simulink model "Pong"  (Simulink 7.0)
settings: Solver=ode4  StartTime=0.0  StopTime=inf  FixedStep=0.001  RelTol=1e-3
undefined symbols (not defined in the file): HIL, qc_get_step_size
libraries: simulink x6, quarc_library x4, vrlib x1
settings Model: Creator=RSamra  LastModifiedBy=colinlea  SimulationMode=external  ExtModeTrigDuration=10000
settings SolverCC: PositivePriorityOrder=on
settings DebuggingCC: MultiTaskDSMMsg=warning  MultiTaskCondExecSysMsg=none  StrictBusMsg=None
settings HardwareCC: TargetHWDeviceType=32-bit Generic
settings RTWCC: SystemTargetFile=quarc_windows.tlc  TemplateMakefile=quarc_default_tmf  Description=QuaRC Win32 Target  ProcessScript=quarc_windows_make_rtw_hook  IncludeERTFirstTime=on
settings STFCustomTargetCC: TargetFcnLib=ansi_tfl_tmw.mat  TargetPreCompLibLocation=C:\DOCUME~1\ALLUSE~1\APPLIC~1\QuaRC\lib\2007b\windows\release  GenFloatMathFcnCalls=ANSI_C  SystemTargetFile=quarc_windows.tlc
settings GRTTargetCC: TargetFcnLib=ansi_tfl_tmw.mat  TargetPreCompLibLocation=C:\DOCUME~1\ALLUSE~1\APPLIC~1\QuaRC\lib\2007b\windows\release  CompOptLevelCompliant=off  MatFileLogging=off  ExtMode=on  ExtModeMexFile=quarc_comm

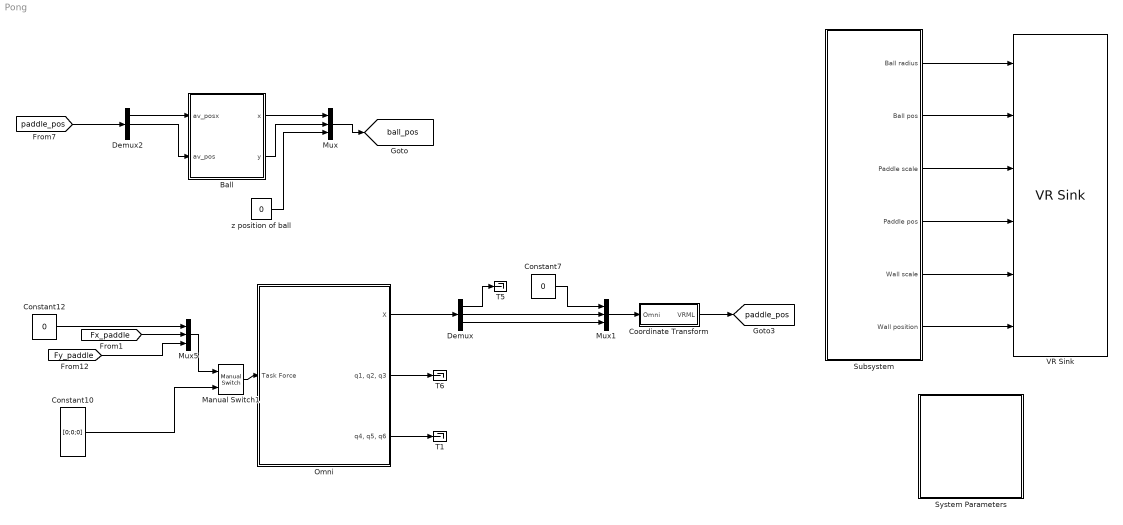
== system Pong ==
  Ball : Subsystem
  Constant10 : Constant  Value=[0;0;0]  VectorParams1D=off  OutDataType=sfix(16)  OutScaling=2^0  SampleTime=0
  Constant12 : Constant  Value=0  VectorParams1D=off  OutDataType=sfix(16)  OutScaling=2^0  SampleTime=0
  Constant7 : Constant  Value=0  VectorParams1D=off  OutDataType=sfix(16)  OutScaling=2^0  SampleTime=0
  Coordinate Transform : Subsystem
  Demux : Demux  Outputs=3
  Demux2 : Demux  Outputs=3
  Manual Switch1 : simulink/Signal Routing/Manual Switch  SystemSampleTime=-1  sw=1  action=0  varsize=off
  Mux : Mux  Inputs=3
  Mux1 : Mux  Inputs=3
  Mux5 : Mux  Inputs=3
  Omni : Subsystem
  Subsystem : Subsystem
  System Parameters : Subsystem
  T1 : Terminator
  T5 : Terminator
  T6 : Terminator
  VR Sink : vrlib/VR Sink  SampleTime=.1  ViewEnable=on  RemoteChange=off  RemoteView=on  FieldsWritten=Ball.scale.3.1.double#Ball.translation.3.1.double#Paddle.scale.3.1.double#Paddle.translation.3.1.double#Walls.scale.3.1.double#Walls.translation.3.1.double  WorldFileName=Pong.WRL  AutoView=on  VideoDimensions=[]  FigureProperties="{'Position', 'Name', 'Viewpoint', 'CameraBound', 'CameraDirection', 'CameraPosition', 'CameraUpVector', 'ZoomFactor', 'Antialiasing', 'Headlight', 'Lighting', 'NavPanel', 'StatusBar', 'ToolBar', 'Textures', 'Transparency', 'Wireframe', 'NavZones', 'NavMode', 'NavSpeed', 'Record2DCompressMethod', 'Record2DCompressQuality', 'Record2D', 'Record2DFileName', 'Record2DFPS'; [-3.0000000000000000e+000  1.1900000000000000e+002  5.7600000000000000e+002  3.8000000000000000e+002], '', '_untitled_1', 'on', [0.0000000000000000e+000  0.0000000000000000e+000 -1.0000000000000000e+000], [0.0000000000000000e+000  0.0000000000000000e+000  0.0000000000000000e+000], [0.0000000000000000e+000  1.0000000000000000e+000  0.0000000000000000e+000], [1.0000000000000000e+000], 'off', 'on', 'on', 'halfbar', 'off', 'on', 'on', 'on', 'off', 'off', 'fly', 'normal', 'auto', [7.5000000000000000e+001], 'off', '%f_anim_%n.avi', [1.5000000000000000e+001]}"
  z position of ball : Constant  Value=0  VectorParams1D=off  OutDataType=sfix(16)  OutScaling=2^0  SampleTime=0
  tag scope: ball_pos=global, paddle_pos=global
  wires:
  Mux/1 -> [ball_pos]
  z position of ball/1 -> Mux/3
  Ball/1(x) -> Mux/1
  Ball/2(y) -> Mux/2
  Constant7/1 -> Mux1/1
  Mux1/1 -> Coordinate Transform/1(Omni)
  Coordinate Transform/1("VRML ") -> [paddle_pos]
  Demux/1 -> T5/1
  Subsystem/1(Ball radius) -> VR Sink/1
  Subsystem/3(Paddle scale) -> VR Sink/3
  Subsystem/5(Wall scale) -> VR Sink/5
  Subsystem/6(Wall position) -> VR Sink/6
  [paddle_pos] -> Demux2/1
  Subsystem/4(Paddle pos) -> VR Sink/4
  Subsystem/2(Ball pos) -> VR Sink/2
  Constant10/1 -> Manual Switch1/2
  Constant12/1 -> Mux5/1
  Mux5/1 -> Manual Switch1/1
  [Fx_paddle] -> Mux5/2
  [Fy_paddle] -> Mux5/3
  Demux2/2 -> Ball/2(av_pos)
  Demux/2 -> Mux1/2
  Demux/3 -> Mux1/3
  Demux2/1 -> Ball/1(av_posx)
  Omni/1(X) -> Demux/1
  Omni/2("q1, q2, q3") -> T6/1
  Omni/3("q4, q5, q6") -> T1/1
  Manual Switch1/1 -> Omni/1(Task Force)

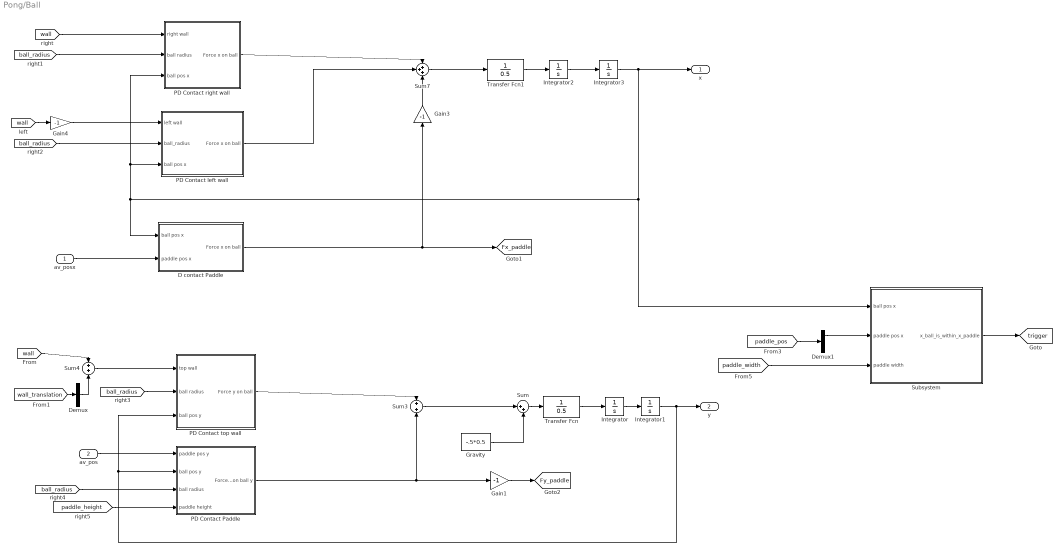
== system Pong/Ball ==
  av_posx : Inport  OutDataType=sfix(16)  OutScaling=2^0
  av_pos : Inport  Port=2  OutDataType=sfix(16)  OutScaling=2^0
  D contact Paddle : Subsystem
  Demux : Demux  Outputs=3
  Demux1 : Demux  Outputs=3
  Gain1 : Gain  Gain=-1  ParameterDataType=sfix(16)  ParameterScaling=2^0  OutDataType=sfix(16)  OutScaling=2^0
  Gain3 : Gain  Orientation=up  Gain=-1  ParameterDataType=sfix(16)  ParameterScaling=2^0  OutDataType=sfix(16)  OutScaling=2^0
  Gain4 : Gain  Gain=-1  ParameterDataType=sfix(16)  ParameterScaling=2^0  OutDataType=sfix(16)  OutScaling=2^0
  Gravity : Constant  Value=-.5*0.5  OutDataType=sfix(16)  OutScaling=2^0  SampleTime=0
  Integrator{,1..3} (4 alike) : Integrator
  PD Contact Paddle : Subsystem
  PD Contact left wall : Subsystem
  PD Contact right wall : Subsystem
  PD Contact top wall : Subsystem
  Subsystem : Subsystem
  Sum : Sum  Inputs=|++  OutDataType=sfix(16)  OutScaling=2^0
  Sum3 : Sum  OutDataType=sfix(16)  OutScaling=2^0
  Sum4 : Sum  OutDataType=sfix(16)  OutScaling=2^0
  Sum7 : Sum  Inputs=+++  OutDataType=sfix(16)  OutScaling=2^0
  Transfer Fcn : TransferFcn  Denominator=[0.5]
  Transfer Fcn1 : TransferFcn  Denominator=[0.5]
  x : Outport
  y : Outport  Port=2
  tag scope: Fx_paddle=global, Fy_paddle=global, trigger=global
  wires:
  Transfer Fcn/1 -> Integrator/1
  Integrator/1 -> Integrator1/1
  Sum/1 -> Transfer Fcn/1
  Gravity/1 -> Sum/2
  Integrator1/1 -> y/1, PD Contact top wall/3(ball pos y), PD Contact Paddle/2(ball pos y)
  PD Contact top wall/1("Force y on ball ") -> Sum3/1
  PD Contact Paddle/1(Force on ball y) -> Sum3/2, Gain1/1
  Sum3/1 -> Sum/1
  Transfer Fcn1/1 -> Integrator2/1
  Integrator2/1 -> Integrator3/1
  Integrator3/1 -> x/1, PD Contact left wall/3(ball pos x), PD Contact right wall/3(ball pos x), D contact Paddle/1(ball pos x), Subsystem/1(ball pos x)
  PD Contact right wall/1(Force x on ball) -> Sum7/1
  PD Contact left wall/1(Force x on ball) -> Sum7/2
  Sum7/1 -> Transfer Fcn1/1
  [wall] -> Sum4/1
  [wall] -> Gain4/1
  [wall] -> PD Contact right wall/1(right wall)
  Gain4/1 -> PD Contact left wall/1(left wall)
  [wall_translation] -> Demux/1
  [paddle_width] -> Subsystem/3(paddle width)
  Subsystem/1(x_ball_is_within_x_paddle) -> [trigger]
  [ball_radius] -> PD Contact left wall/2(ball_radius)
  Gain1/1 -> [Fy_paddle]
  Demux/2 -> Sum4/2
  [ball_radius] -> PD Contact top wall/2(ball radius)
  Sum4/1 -> PD Contact top wall/1(top wall)
  av_pos/1 -> PD Contact Paddle/1(paddle pos y)
  [ball_radius] -> PD Contact Paddle/3(ball radius)
  [paddle_height] -> PD Contact Paddle/4(paddle height)
  [ball_radius] -> PD Contact right wall/2(ball radius)
  Gain3/1 -> Sum7/3
  av_posx/1 -> D contact Paddle/2(paddle pos x)
  D contact Paddle/1("Force x on ball ") -> Gain3/1, [Fx_paddle]
  [paddle_pos] -> Demux1/1
  Demux1/1 -> Subsystem/2(paddle pos x)

== system Pong/Coordinate Transform ==
  Omni : Inport  Orientation=down
  Demux1 : Demux  Outputs=3
  Mux : Mux  Inputs=3
  "VRML " : Outport
  wires:
  Omni/1 -> Demux1/1
  Mux/1 -> "VRML "/1
  Demux1/1 -> Mux/3
  Demux1/3 -> Mux/2
  Demux1/2 -> Mux/1

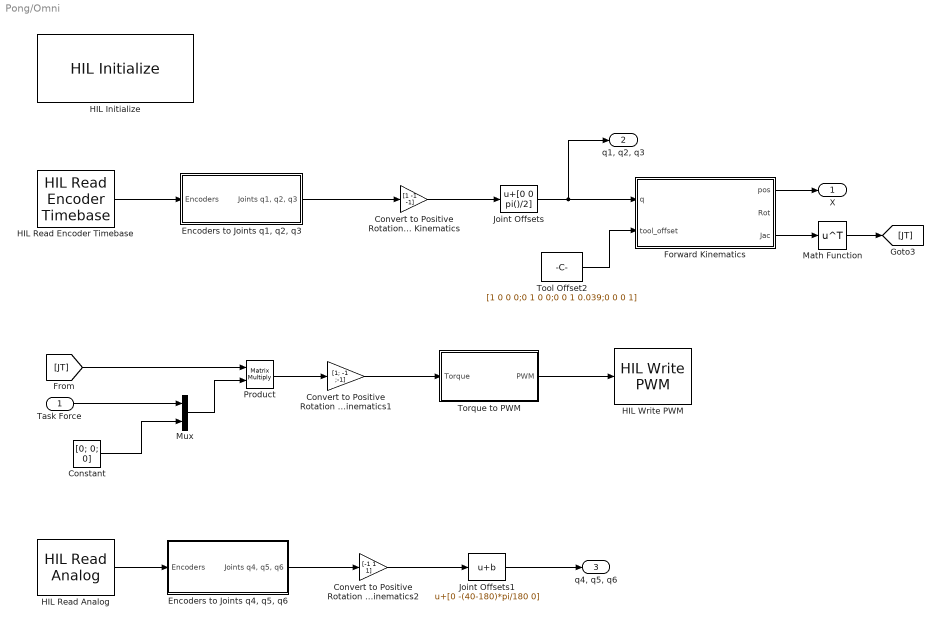
== system Pong/Omni ==
  Task Force : Inport
  Constant : Constant  Value=[0; 0; 0]  VectorParams1D=off  OutDataType=sfix(16)  OutScaling=2^0
  Convert to Positive Rotation Convension Used in Kinematics : Gain  Gain=[1 -1 -1]  ParameterDataType=sfix(16)  ParameterScaling=2^0  OutDataType=sfix(16)  OutScaling=2^0
  Convert to Positive Rotation Convension Used in Kinematics1 : Gain  Gain=[1; -1 ;-1]  ParameterDataType=sfix(16)  ParameterScaling=2^0  OutDataType=sfix(16)  OutScaling=2^0
  Convert to Positive Rotation Convension Used in Kinematics2 : Gain  Gain=[-1 1 1]  ParameterDataType=sfix(16)  ParameterScaling=2^0  OutDataType=sfix(16)  OutScaling=2^0
  "Encoders to Joints q1, q2, q3" : Subsystem
  "Encoders to Joints q4, q5, q6" : Subsystem
  "Forward Kinematics " : Stateflow chart
  HIL Initialize : quarc_library/Data Acquisition/Generic/Configuration/HIL Initialize  object_name=HIL-1  board_type=phantom_omni  board_number=0  active=on  hardware_clocks=[]  clock_modes=[]  set_clock_params_at_start=off  set_clock_params_at_switch_in=off  analog_input_channels=0:1  analog_input_maximums=10  analog_input_minimums=-10  set_analog_input_params_at_start=off  set_analog_input_params_at_switch_in=off  analog_output_channels=[]  analog_output_maximums=[]  analog_output_minimums=[]  initial_analog_outputs=[]  final_analog_outputs=[]  watchdog_analog_outputs=0  set_analog_output_params_at_start=off  set_analog_output_params_at_switch_in=off  set_analog_outputs_at_start=off  set_analog_outputs_at_switch_in=off  set_analog_outputs_at_terminate=off  set_analog_outputs_at_switch_out=off  set_analog_outputs_on_watchdog=off  digital_input_channels=[]  digital_output_channels=[]  initial_digital_outputs=[]  final_digital_outputs=[]  watchdog_digital_outputs=0  set_digital_outputs_at_start=off  set_digital_outputs_at_switch_in=off  set_digital_outputs_at_terminate=off  set_digital_outputs_at_switch_out=off  set_digital_outputs_on_watchdog=off  encoder_channels=0:2  quadrature=[]  encoder_filter_frequency=[]  initial_encoder_counts=0  set_encoder_params_at_start=off  set_encoder_params_at_switch_in=off  set_encoder_counts_at_start=off  set_encoder_counts_at_switch_in=off  pwm_channels=0:2  pwm_modes=[]  pwm_frequency=[]  initial_pwm_outputs=0  final_pwm_outputs=0  watchdog_pwm_outputs=0  set_pwm_params_at_start=off  set_pwm_params_at_switch_in=off  set_pwm_outputs_at_start=on  set_pwm_outputs_at_switch_in=off  set_pwm_outputs_at_terminate=on  set_pwm_outputs_at_switch_out=off  set_pwm_outputs_on_watchdog=off  other_output_channels=[]  initial_other_outputs=[]  final_other_outputs=[]  watchdog_other_outputs=0  set_other_outputs_at_start=off  set_other_outputs_at_switch_in=off  set_other_outputs_at_terminate=off  set_other_outputs_at_switch_out=off  set_other_outputs_on_watchdog=off
  HIL Read Analog : quarc_library/Data Acquisition/Generic/Immediate I//O/HIL Read Analog  object_name=HIL-1  channels=[0:2]  sample_time=qc_get_step_size  active=on  vector_output=on
  HIL Read Encoder Timebase : quarc_library/Data Acquisition/Generic/Timebases/HIL Read Encoder Timebase  object_name=HIL-1  clock=0  channels=0:2  samples_in_buffer=max(ceil(1/qc_get_step_size), 1)  active=on  vector_output=on  data_type_mode=Inherit via back propagation  data_type=double
  HIL Write PWM : quarc_library/Data Acquisition/Generic/Immediate I//O/HIL Write PWM  object_name=HIL-1  channels=0:2  sample_time=-1  active=off  vector_input=on
      settings: AttributesFormatString=(%<object_name>)
  Joint Offsets : Bias  Bias=[0 0 pi()/2]
  Joint Offsets1 : Bias  Bias=[0 -(40-180)*pi/180 0]  SaturateOnIntegerOverflow=on
  Math Function : Math  Operator=transpose  OutDataType=sfix(16)  OutScaling=2^0  SaturateOnIntegerOverflow=on
  Mux : Mux  Inputs=2
  Product : Product  Multiplication=Matrix(*)  OutDataType=sfix(16)  OutScaling=2^0  RndMeth=Zero
  Tool Offset2 : Constant  Value=[1 0 0 0;0 1 0 0;0 0 1 0.039;0 0 0 1]  VectorParams1D=off  OutDataType=sfix(16)  OutScaling=2^0
  Torque to PWM : Subsystem
  X : Outport
  "q1, q2, q3" : Outport  Port=2
  "q4, q5, q6" : Outport  Port=3
  wires:
  Tool Offset2/1 -> "Forward Kinematics "/2(tool_offset)
  Math Function/1 -> [JT]
  "Forward Kinematics "/3(Jac) -> Math Function/1
  [JT] -> Product/1
  Torque to PWM/1(PWM) -> HIL Write PWM/1
  "Forward Kinematics "/1(pos) -> X/1
  Constant/1 -> Mux/2
  Task Force/1 -> Mux/1
  Mux/1 -> Product/2
  "Encoders to Joints q1, q2, q3"/1("Joints q1, q2, q3") -> Convert to Positive Rotation Convension Used in Kinematics/1
  Convert to Positive Rotation Convension Used in Kinematics/1 -> Joint Offsets/1
  Convert to Positive Rotation Convension Used in Kinematics1/1 -> Torque to PWM/1(Torque)
  Product/1 -> Convert to Positive Rotation Convension Used in Kinematics1/1
  Joint Offsets/1 -> "Forward Kinematics "/1(q), "q1, q2, q3"/1
  HIL Read Encoder Timebase/1 -> "Encoders to Joints q1, q2, q3"/1(Encoders)
  HIL Read Analog/1 -> "Encoders to Joints q4, q5, q6"/1(Encoders)
  Convert to Positive Rotation Convension Used in Kinematics2/1 -> Joint Offsets1/1
  "Encoders to Joints q4, q5, q6"/1("Joints q4, q5, q6") -> Convert to Positive Rotation Convension Used in Kinematics2/1
  Joint Offsets1/1 -> "q4, q5, q6"/1

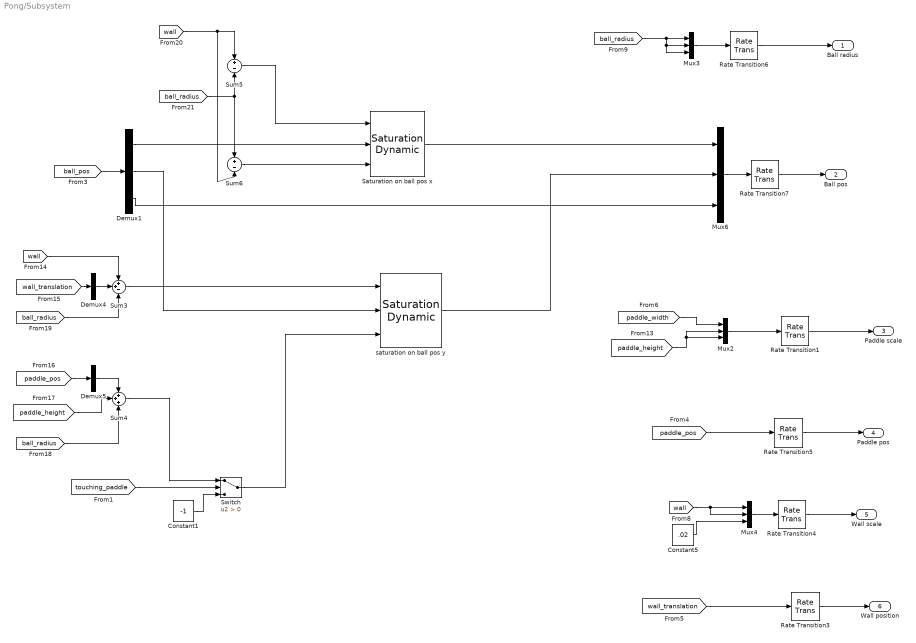
== system Pong/Subsystem ==
  Constant1 : Constant  Value=-1  OutDataType=sfix(16)  OutScaling=2^0
  Constant5 : Constant  Value=.02  VectorParams1D=off  OutDataType=sfix(16)  OutScaling=2^0  SampleTime=0
  Demux1 : Demux  Outputs=3
  Demux4 : Demux  Outputs=3
  Demux5 : Demux  Outputs=3
  Mux{2..4,6} (4 alike) : Mux  Inputs=3
  Rate Transition{1,3..7} (6 alike) : RateTransition
  Saturation on ball pos x : simulink/Discontinuities/Saturation Dynamic  SystemSampleTime=-1  OutMin=[]  OutMax=[]  OutDataTypeStr=Inherit: Same as second input  OutDataType=sfix(16)  OutScaling=2^-10  DoSatur=off
  Sum3 : Sum  Inputs=++-  OutDataType=sfix(16)  OutScaling=2^0
  Sum4 : Sum  Inputs=+++  OutDataType=sfix(16)  OutScaling=2^0
  Sum5 : Sum  Inputs=+-  OutDataType=sfix(16)  OutScaling=2^0
  Sum6 : Sum  Inputs=+-  OutDataType=sfix(16)  OutScaling=2^0
  Switch : Switch  Criteria=u2 > Threshold
  saturation on ball pos y : simulink/Discontinuities/Saturation Dynamic  SystemSampleTime=-1  OutMin=[]  OutMax=[]  OutDataTypeStr=Inherit: Same as second input  OutDataType=sfix(16)  OutScaling=2^-10  DoSatur=off
  Ball radius : Outport
  Ball pos : Outport  Port=2
  Paddle scale : Outport  Port=3
  Paddle pos : Outport  Port=4
  Wall scale : Outport  Port=5
  Wall position : Outport  Port=6
  wires:
  [paddle_width] -> Mux2/1
  [paddle_height] -> Mux2/2, Mux2/3
  [ball_radius] -> Mux3/1, Mux3/2, Mux3/3
  Mux4/1 -> Rate Transition4/1
  Mux2/1 -> Rate Transition1/1
  Mux3/1 -> Rate Transition6/1
  [wall] -> Mux4/1, Mux4/2
  Constant5/1 -> Mux4/3
  [paddle_pos] -> Rate Transition5/1
  [wall_translation] -> Rate Transition3/1
  [ball_pos] -> Demux1/1
  Mux6/1 -> Rate Transition7/1
  Demux1/3 -> Mux6/3
  Demux1/2 -> saturation on ball pos y/2
  saturation on ball pos y/1 -> Mux6/2
  [wall_translation] -> Demux4/1
  [wall] -> Sum3/1
  Demux4/2 -> Sum3/2
  Sum3/1 -> saturation on ball pos y/1
  [paddle_pos] -> Demux5/1
  Demux5/2 -> Sum4/1
  [paddle_height] -> Sum4/2
  [ball_radius] -> Sum4/3
  [ball_radius] -> Sum3/3
  Demux1/1 -> Saturation on ball pos x/2
  Saturation on ball pos x/1 -> Mux6/1
  [wall] -> Sum5/1, Sum6/2
  [ball_radius] -> Sum5/2, Sum6/1
  Sum5/1 -> Saturation on ball pos x/1
  Rate Transition6/1 -> Ball radius/1
  Rate Transition7/1 -> Ball pos/1
  Rate Transition1/1 -> Paddle scale/1
  Rate Transition5/1 -> Paddle pos/1
  Rate Transition4/1 -> Wall scale/1
  Rate Transition3/1 -> Wall position/1
  Sum6/1 -> Saturation on ball pos x/3
  Switch/1 -> saturation on ball pos y/3
  [touching_paddle] -> Switch/2
  Sum4/1 -> Switch/1
  Constant1/1 -> Switch/3

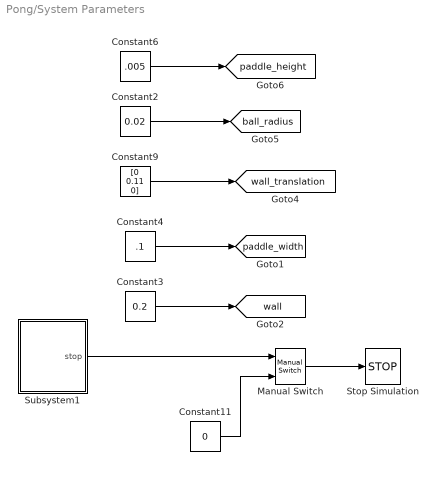
== system Pong/System Parameters ==
  Constant11 : Constant  Value=0  OutDataType=sfix(16)  OutScaling=2^0  SampleTime=0
  Constant2 : Constant  Value=0.02  VectorParams1D=off  OutDataType=sfix(16)  OutScaling=2^0
  Constant3 : Constant  Value=0.2  OutDataType=sfix(16)  OutScaling=2^0  SampleTime=0
  Constant4 : Constant  Value=.1  VectorParams1D=off  OutDataType=sfix(16)  OutScaling=2^0  SampleTime=0
  Constant6 : Constant  Value=.005  VectorParams1D=off  OutDataType=sfix(16)  OutScaling=2^0  SampleTime=0
  Constant9 : Constant  Value=[0 0.11 0]  VectorParams1D=off  OutDataType=sfix(16)  OutScaling=2^0  SampleTime=0
  Manual Switch : simulink/Signal Routing/Manual Switch  SystemSampleTime=-1  sw=1  action=0  varsize=off
  Stop Simulation : Stop
  Subsystem1 : Subsystem
  tag scope: ball_radius=global, paddle_height=global, paddle_width=global, wall=global, wall_translation=global
  wires:
  Constant4/1 -> [paddle_width]
  Constant3/1 -> [wall]
  Constant9/1 -> [wall_translation]
  Manual Switch/1 -> Stop Simulation/1
  Subsystem1/1(stop) -> Manual Switch/1
  Constant11/1 -> Manual Switch/2
  Constant2/1 -> [ball_radius]
  Constant6/1 -> [paddle_height]

== system Pong/Ball/D contact Paddle ==
  ball pos x : Inport
  paddle pos x : Inport  Port=2
  Compare To Constant1 : simulink/Logic and Bit Operations/Compare To Constant  SystemSampleTime=-1  relop=~=  const=0  LogicOutDataTypeMode=uint8  ZeroCross=off
  Logical Operator2 : Logic  AllPortsSameDT=off  OutDataTypeMode=boolean
  Subsystem5 : Subsystem
  Sum10 : Sum  Inputs=-+  OutDataType=sfix(16)  OutScaling=2^0
  Switch4 : Switch  Criteria=u2 > Threshold
  non contact Force4 : Constant  Value=0  VectorParams1D=off  OutDataType=sfix(16)  OutScaling=2^0  SampleTime=0
  "Force x on ball " : Outport
  wires:
  Sum10/1 -> Compare To Constant1/1, Subsystem5/1(In1)
  Compare To Constant1/1 -> Logical Operator2/1
  Logical Operator2/1 -> Switch4/2
  non contact Force4/1 -> Switch4/3
  Subsystem5/1(Fball) -> Switch4/1
  ball pos x/1 -> Sum10/1
  Switch4/1 -> "Force x on ball "/1
  paddle pos x/1 -> Sum10/2
  [touching_paddle] -> Logical Operator2/2

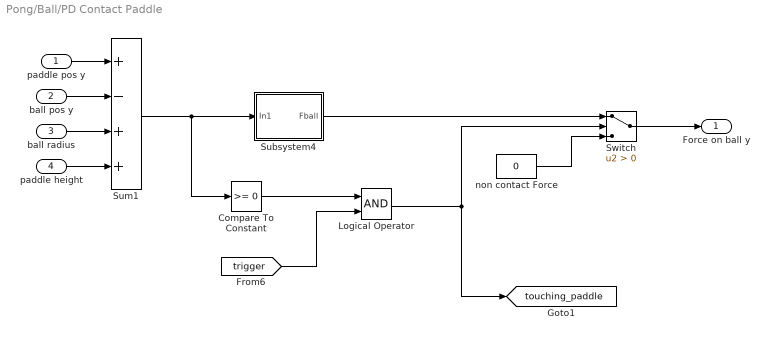
== system Pong/Ball/PD Contact Paddle ==
  paddle pos y : Inport
  ball pos y : Inport  Port=2
  ball radius : Inport  Port=3
  paddle height : Inport  Port=4
  Compare To Constant : simulink/Logic and Bit Operations/Compare To Constant  SystemSampleTime=-1  relop=>=  const=0  LogicOutDataTypeMode=uint8  ZeroCross=off
  Logical Operator : Logic  AllPortsSameDT=off  OutDataTypeMode=boolean
  Subsystem4 : Subsystem
  Sum1 : Sum  Inputs=+-++  OutDataType=sfix(16)  OutScaling=2^0
  Switch : Switch  Criteria=u2 > Threshold
  non contact Force : Constant  Value=0  VectorParams1D=off  OutDataType=sfix(16)  OutScaling=2^0  SampleTime=0
  Force on ball y : Outport
  tag scope: touching_paddle=global
  wires:
  Sum1/1 -> Subsystem4/1(In1), Compare To Constant/1
  Compare To Constant/1 -> Logical Operator/1
  [trigger] -> Logical Operator/2
  Logical Operator/1 -> Switch/2, [touching_paddle]
  Subsystem4/1(Fball) -> Switch/1
  non contact Force/1 -> Switch/3
  ball pos y/1 -> Sum1/2
  paddle pos y/1 -> Sum1/1
  Switch/1 -> Force on ball y/1
  ball radius/1 -> Sum1/3
  paddle height/1 -> Sum1/4

== system Pong/Ball/PD Contact left wall ==
  left wall : Inport
  ball_radius : Inport  Port=2
  ball pos x : Inport  Port=3
  Subsystem1 : Subsystem
  Sum5 : Sum  Inputs=++-  OutDataType=sfix(16)  OutScaling=2^0
  Switch2 : Switch
  non contact Force2 : Constant  Value=0  VectorParams1D=off  OutDataType=sfix(16)  OutScaling=2^0  SampleTime=0
  Force x on ball : Outport
  wires:
  non contact Force2/1 -> Switch2/3
  Subsystem1/1(Fball) -> Switch2/1
  Sum5/1 -> Subsystem1/1(In1), Switch2/2
  ball_radius/1 -> Sum5/2
  left wall/1 -> Sum5/1
  Switch2/1 -> Force x on ball/1
  ball pos x/1 -> Sum5/3

== system Pong/Ball/PD Contact right wall ==
  right wall : Inport
  ball radius : Inport  Port=2
  ball pos x : Inport  Port=3
  Subsystem2 : Subsystem
  Sum6 : Sum  Inputs=+--  OutDataType=sfix(16)  OutScaling=2^0
  Switch3 : Switch
  non contact Force3 : Constant  Value=0  VectorParams1D=off  OutDataType=sfix(16)  OutScaling=2^0  SampleTime=0
  Force x on ball : Outport
  wires:
  non contact Force3/1 -> Switch3/1
  Sum6/1 -> Switch3/2, Subsystem2/1(In1)
  Subsystem2/1(Fball) -> Switch3/3
  Switch3/1 -> Force x on ball/1
  right wall/1 -> Sum6/1
  ball radius/1 -> Sum6/2
  ball pos x/1 -> Sum6/3

== system Pong/Ball/PD Contact top wall ==
  top wall : Inport
  ball radius : Inport  Port=2
  ball pos y : Inport  Port=3
  Subsystem3 : Subsystem
  Sum2 : Sum  Inputs=+--  OutDataType=sfix(16)  OutScaling=2^0
  Switch1 : Switch
  non contact Force1 : Constant  Value=0  VectorParams1D=off  OutDataType=sfix(16)  OutScaling=2^0  SampleTime=0
  "Force y on ball " : Outport
  wires:
  Subsystem3/1(Fball) -> Switch1/3
  non contact Force1/1 -> Switch1/1
  ball pos y/1 -> Sum2/3
  Switch1/1 -> "Force y on ball "/1
  top wall/1 -> Sum2/1
  ball radius/1 -> Sum2/2
  Sum2/1 -> Subsystem3/1(In1), Switch1/2

== system Pong/Ball/Subsystem ==
  ball pos x : Inport
  paddle pos x : Inport  Port=2
  paddle width : Inport  Port=3
  Logical Operator1 : Logic  AllPortsSameDT=off  OutDataTypeMode=boolean
  Relational Operator : RelationalOperator  Operator=<=  LogicOutDataTypeMode=boolean
  Relational Operator1 : RelationalOperator  LogicOutDataTypeMode=boolean
  Sum8 : Sum  OutDataType=sfix(16)  OutScaling=2^0
  Sum9 : Sum  Inputs=-+  OutDataType=sfix(16)  OutScaling=2^0
  x_ball_is_within_x_paddle : Outport
  wires:
  Sum8/1 -> Relational Operator/2
  Sum9/1 -> Relational Operator1/2
  Relational Operator/1 -> Logical Operator1/1
  Relational Operator1/1 -> Logical Operator1/2
  ball pos x/1 -> Relational Operator/1, Relational Operator1/1
  paddle pos x/1 -> Sum8/1, Sum9/2
  paddle width/1 -> Sum8/2, Sum9/1
  Logical Operator1/1 -> x_ball_is_within_x_paddle/1

== system Pong/Omni/Encoders to Joints q1, q2, q3 ==
  Encoders : Inport
  Bias1 : Bias  Bias=[0 -659 -910]
  Embedded MATLAB Function : Stateflow chart
  Encoder : Gain  Gain=2*pi/2048  ParameterDataType=sfix(16)  ParameterScaling=2^0  OutDataType=sfix(16)  OutScaling=2^0
  Gear Ratio : Gain  Gain=1./[7.461 -7.519 7.529]  ParameterDataType=sfix(16)  ParameterScaling=2^0  OutDataType=sfix(16)  OutScaling=2^0
  "Joints q1, q2, q3" : Outport
  wires:
  Embedded MATLAB Function/1(q) -> "Joints q1, q2, q3"/1
  Encoders/1 -> Bias1/1
  Encoder/1 -> Gear Ratio/1
  Gear Ratio/1 -> Embedded MATLAB Function/1(m)
  Bias1/1 -> Encoder/1

== system Pong/Omni/Encoders to Joints q4, q5, q6 ==
  Encoders : Inport
  Bias1 : Bias  Bias=[-2048 -2654 -2048]
  Gain2 : Gain  Gain=[2*pi()/4915 2*pi()/4096 2*pi()/4915]  ParameterDataType=sfix(16)  ParameterScaling=2^0  OutDataType=sfix(16)  OutScaling=2^0
  "Joints q4, q5, q6" : Outport
  wires:
  Bias1/1 -> Gain2/1
  Encoders/1 -> Bias1/1
  Gain2/1 -> "Joints q4, q5, q6"/1

== system Pong/Omni/Torque to PWM ==
  Torque : Inport
  Gear Ratio1 : Gain  Gain=1./[7.461 -7.519 7.529]  ParameterDataType=sfix(16)  ParameterScaling=2^0  OutDataType=sfix(16)  OutScaling=2^0
  Joint Torque to Motor Torque : Stateflow chart
  Kt : Gain  Gain=1./38.526e-3  ParameterDataType=sfix(16)  ParameterScaling=2^0  OutDataType=sfix(16)  OutScaling=2^0
  Saturation : Saturate  UpperLimit=1.6  LowerLimit=-1.6
  Smart Saturation : Stateflow chart
  PWM : Outport
  wires:
  Torque/1 -> Joint Torque to Motor Torque/1(t)
  Smart Saturation/1(y) -> PWM/1
  Saturation/1 -> Smart Saturation/1(u)
  Kt/1 -> Saturation/1
  Gear Ratio1/1 -> Kt/1
  Joint Torque to Motor Torque/1(y) -> Gear Ratio1/1

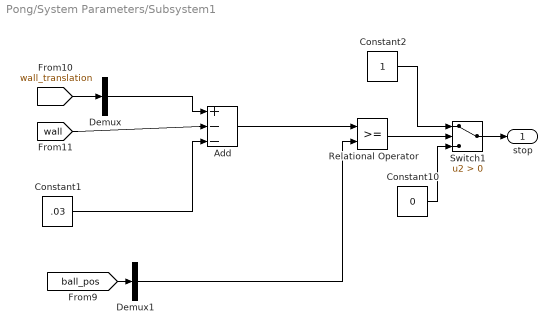
== system Pong/System Parameters/Subsystem1 ==
  Add : Sum  Inputs=|+--  OutDataType=sfix(16)  OutScaling=2^-10
  Constant1 : Constant  Value=.03  OutDataType=sfix(16)  OutScaling=2^0  SampleTime=0
  Constant10 : Constant  Value=0  OutDataType=sfix(16)  OutScaling=2^0  SampleTime=0
  Constant2 : Constant  OutDataType=sfix(16)  OutScaling=2^0  SampleTime=0
  Demux : Demux  Outputs=3
  Demux1 : Demux  Outputs=3
  Relational Operator : RelationalOperator  LogicOutDataTypeMode=boolean
  Switch1 : Switch  Criteria=u2 > Threshold
  stop : Outport
  wires:
  [wall] -> Add/2
  Add/1 -> Relational Operator/1
  Relational Operator/1 -> Switch1/2
  Constant2/1 -> Switch1/1
  Constant10/1 -> Switch1/3
  Switch1/1 -> stop/1
  [wall_translation] -> Demux/1
  [ball_pos] -> Demux1/1
  Demux1/2 -> Relational Operator/2
  Demux/2 -> Add/1
  Constant1/1 -> Add/3

== system Pong/Ball/D contact Paddle/Subsystem5 ==
  In1 : Inport
  2nd Order Filter Input ICs : Subsystem
  Gain1 : Gain  Gain=2  ParameterDataType=sfix(16)  ParameterScaling=2^0  OutDataType=sfix(16)  OutScaling=2^0
  Gain3 : Gain  Gain=0  ParameterDataType=sfix(16)  ParameterScaling=2^0  OutDataType=sfix(16)  OutScaling=2^0
  Subtract : Sum  Inputs=+-  OutDataType=sfix(16)  OutScaling=2^-10
  Wn : Constant  Value=200  VectorParams1D=off  OutDataType=sfix(16)  OutScaling=2^0  SampleTime=0
  z : Constant  VectorParams1D=off  OutDataType=sfix(16)  OutScaling=2^0  SampleTime=0
  Fball : Outport
  wires:
  Subtract/1 -> Fball/1
  Gain1/1 -> Subtract/2
  2nd Order Filter Input ICs/2(Out_dot) -> Gain1/1
  Gain3/1 -> Subtract/1
  In1/1 -> Gain3/1, 2nd Order Filter Input ICs/1(In)
  z/1 -> 2nd Order Filter Input ICs/3(z)
  Wn/1 -> 2nd Order Filter Input ICs/2(Wn)

== system Pong/Ball/PD Contact Paddle/Subsystem4 ==
  In1 : Inport
  2nd Order Filter Input ICs : Subsystem
  Gain1 : Gain  Gain=.01  ParameterDataType=sfix(16)  ParameterScaling=2^0  OutDataType=sfix(16)  OutScaling=2^0
  Gain3 : Gain  Gain=500  ParameterDataType=sfix(16)  ParameterScaling=2^0  OutDataType=sfix(16)  OutScaling=2^0
  Subtract : Sum  Inputs=+-  OutDataType=sfix(16)  OutScaling=2^-10
  Wn : Constant  Value=200  VectorParams1D=off  OutDataType=sfix(16)  OutScaling=2^0  SampleTime=0
  z : Constant  VectorParams1D=off  OutDataType=sfix(16)  OutScaling=2^0  SampleTime=0
  Fball : Outport
  wires:
  Subtract/1 -> Fball/1
  Gain1/1 -> Subtract/2
  2nd Order Filter Input ICs/2(Out_dot) -> Gain1/1
  Gain3/1 -> Subtract/1
  In1/1 -> Gain3/1, 2nd Order Filter Input ICs/1(In)
  z/1 -> 2nd Order Filter Input ICs/3(z)
  Wn/1 -> 2nd Order Filter Input ICs/2(Wn)

== system Pong/Ball/PD Contact left wall/Subsystem1 ==
  In1 : Inport
  2nd Order Filter Input ICs : Subsystem
  Gain1 : Gain  Gain=.01  ParameterDataType=sfix(16)  ParameterScaling=2^0  OutDataType=sfix(16)  OutScaling=2^0
  Gain3 : Gain  Gain=500  ParameterDataType=sfix(16)  ParameterScaling=2^0  OutDataType=sfix(16)  OutScaling=2^0
  Subtract : Sum  Inputs=+-  OutDataType=sfix(16)  OutScaling=2^-10
  Wn : Constant  Value=200  VectorParams1D=off  OutDataType=sfix(16)  OutScaling=2^0  SampleTime=0
  z : Constant  VectorParams1D=off  OutDataType=sfix(16)  OutScaling=2^0  SampleTime=0
  Fball : Outport
  wires:
  Subtract/1 -> Fball/1
  Gain1/1 -> Subtract/2
  2nd Order Filter Input ICs/2(Out_dot) -> Gain1/1
  Gain3/1 -> Subtract/1
  In1/1 -> Gain3/1, 2nd Order Filter Input ICs/1(In)
  z/1 -> 2nd Order Filter Input ICs/3(z)
  Wn/1 -> 2nd Order Filter Input ICs/2(Wn)

== system Pong/Ball/PD Contact right wall/Subsystem2 ==
  In1 : Inport
  2nd Order Filter Input ICs : Subsystem
  Gain1 : Gain  Gain=.01  ParameterDataType=sfix(16)  ParameterScaling=2^0  OutDataType=sfix(16)  OutScaling=2^0
  Gain3 : Gain  Gain=500  ParameterDataType=sfix(16)  ParameterScaling=2^0  OutDataType=sfix(16)  OutScaling=2^0
  Subtract : Sum  Inputs=+-  OutDataType=sfix(16)  OutScaling=2^-10
  Wn : Constant  Value=200  VectorParams1D=off  OutDataType=sfix(16)  OutScaling=2^0  SampleTime=0
  z : Constant  VectorParams1D=off  OutDataType=sfix(16)  OutScaling=2^0  SampleTime=0
  Fball : Outport
  wires:
  Wn/1 -> 2nd Order Filter Input ICs/2(Wn)
  z/1 -> 2nd Order Filter Input ICs/3(z)
  In1/1 -> 2nd Order Filter Input ICs/1(In), Gain3/1
  Gain3/1 -> Subtract/1
  2nd Order Filter Input ICs/2(Out_dot) -> Gain1/1
  Gain1/1 -> Subtract/2
  Subtract/1 -> Fball/1

== system Pong/Ball/PD Contact top wall/Subsystem3 ==
  In1 : Inport
  2nd Order Filter Input ICs : Subsystem
  Gain1 : Gain  Gain=.01  ParameterDataType=sfix(16)  ParameterScaling=2^0  OutDataType=sfix(16)  OutScaling=2^0
  Gain3 : Gain  Gain=500  ParameterDataType=sfix(16)  ParameterScaling=2^0  OutDataType=sfix(16)  OutScaling=2^0
  Subtract : Sum  Inputs=+-  OutDataType=sfix(16)  OutScaling=2^-10
  Wn : Constant  Value=200  VectorParams1D=off  OutDataType=sfix(16)  OutScaling=2^0  SampleTime=0
  z : Constant  VectorParams1D=off  OutDataType=sfix(16)  OutScaling=2^0  SampleTime=0
  Fball : Outport
  wires:
  Wn/1 -> 2nd Order Filter Input ICs/2(Wn)
  z/1 -> 2nd Order Filter Input ICs/3(z)
  In1/1 -> 2nd Order Filter Input ICs/1(In), Gain3/1
  Gain3/1 -> Subtract/1
  2nd Order Filter Input ICs/2(Out_dot) -> Gain1/1
  Gain1/1 -> Subtract/2
  Subtract/1 -> Fball/1

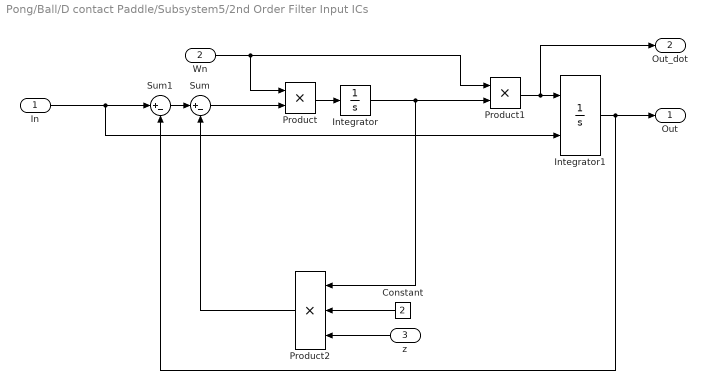
== system Pong/Ball/D contact Paddle/Subsystem5/2nd Order Filter Input ICs ==
  In : Inport  OutDataType=sfix(16)  OutScaling=2^0
  Wn : Inport  Port=2  OutDataType=sfix(16)  OutScaling=2^0
  z : Inport  Orientation=left  Port=3  OutDataType=sfix(16)  OutScaling=2^0
  Constant : Constant  Orientation=left  Value=2  OutDataType=sfix(16)  OutScaling=2^0
  Integrator : Integrator
  Integrator1 : Integrator  InitialConditionSource=external
  Product : Product  OutDataType=sfix(16)  OutScaling=2^0  RndMeth=Zero
  Product1 : Product  OutDataType=sfix(16)  OutScaling=2^0  RndMeth=Zero
  Product2 : Product  Orientation=left  Inputs=3  OutDataType=sfix(16)  OutScaling=2^0  RndMeth=Zero
  Sum : Sum  Inputs=|+-  OutDataType=sfix(16)  OutScaling=2^0
  Sum1 : Sum  Inputs=|+-  OutDataType=sfix(16)  OutScaling=2^0
  Out : Outport  OutDataType=sfix(16)  OutScaling=2^0
  Out_dot : Outport  Port=2  OutDataType=sfix(16)  OutScaling=2^0
  wires:
  Constant/1 -> Product2/2
  z/1 -> Product2/3
  Product2/1 -> Sum/2
  In/1 -> Integrator1/2, Sum1/1
  Sum1/1 -> Sum/1
  Integrator1/1 -> Out/1, Sum1/2
  Integrator/1 -> Product2/1, Product1/2
  Product1/1 -> Out_dot/1, Integrator1/1
  Wn/1 -> Product1/1, Product/1
  Sum/1 -> Product/2
  Product/1 -> Integrator/1

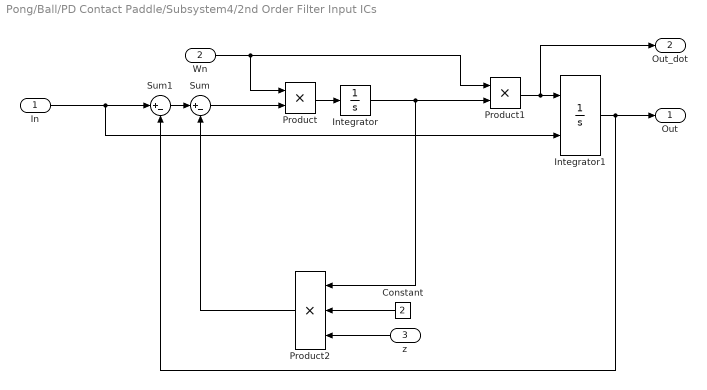
== system Pong/Ball/PD Contact Paddle/Subsystem4/2nd Order Filter Input ICs ==
  In : Inport  OutDataType=sfix(16)  OutScaling=2^0
  Wn : Inport  Port=2  OutDataType=sfix(16)  OutScaling=2^0
  z : Inport  Orientation=left  Port=3  OutDataType=sfix(16)  OutScaling=2^0
  Constant : Constant  Orientation=left  Value=2  OutDataType=sfix(16)  OutScaling=2^0
  Integrator : Integrator
  Integrator1 : Integrator  InitialConditionSource=external
  Product : Product  OutDataType=sfix(16)  OutScaling=2^0  RndMeth=Zero
  Product1 : Product  OutDataType=sfix(16)  OutScaling=2^0  RndMeth=Zero
  Product2 : Product  Orientation=left  Inputs=3  OutDataType=sfix(16)  OutScaling=2^0  RndMeth=Zero
  Sum : Sum  Inputs=|+-  OutDataType=sfix(16)  OutScaling=2^0
  Sum1 : Sum  Inputs=|+-  OutDataType=sfix(16)  OutScaling=2^0
  Out : Outport  OutDataType=sfix(16)  OutScaling=2^0
  Out_dot : Outport  Port=2  OutDataType=sfix(16)  OutScaling=2^0
  wires:
  Constant/1 -> Product2/2
  z/1 -> Product2/3
  Product2/1 -> Sum/2
  In/1 -> Integrator1/2, Sum1/1
  Sum1/1 -> Sum/1
  Integrator1/1 -> Out/1, Sum1/2
  Integrator/1 -> Product2/1, Product1/2
  Product1/1 -> Out_dot/1, Integrator1/1
  Wn/1 -> Product1/1, Product/1
  Sum/1 -> Product/2
  Product/1 -> Integrator/1

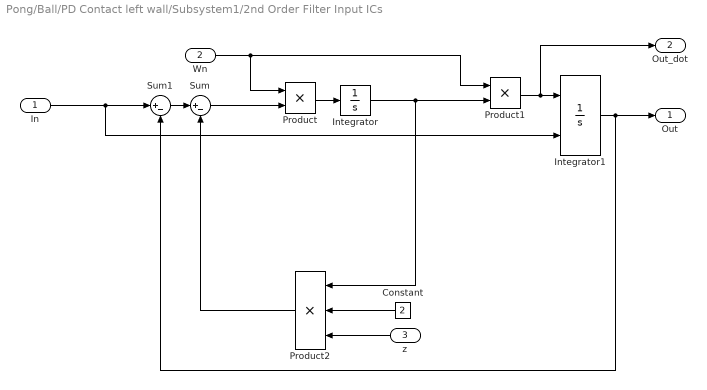
== system Pong/Ball/PD Contact left wall/Subsystem1/2nd Order Filter Input ICs ==
  In : Inport  OutDataType=sfix(16)  OutScaling=2^0
  Wn : Inport  Port=2  OutDataType=sfix(16)  OutScaling=2^0
  z : Inport  Orientation=left  Port=3  OutDataType=sfix(16)  OutScaling=2^0
  Constant : Constant  Orientation=left  Value=2  OutDataType=sfix(16)  OutScaling=2^0
  Integrator : Integrator
  Integrator1 : Integrator  InitialConditionSource=external
  Product : Product  OutDataType=sfix(16)  OutScaling=2^0  RndMeth=Zero
  Product1 : Product  OutDataType=sfix(16)  OutScaling=2^0  RndMeth=Zero
  Product2 : Product  Orientation=left  Inputs=3  OutDataType=sfix(16)  OutScaling=2^0  RndMeth=Zero
  Sum : Sum  Inputs=|+-  OutDataType=sfix(16)  OutScaling=2^0
  Sum1 : Sum  Inputs=|+-  OutDataType=sfix(16)  OutScaling=2^0
  Out : Outport  OutDataType=sfix(16)  OutScaling=2^0
  Out_dot : Outport  Port=2  OutDataType=sfix(16)  OutScaling=2^0
  wires:
  Constant/1 -> Product2/2
  z/1 -> Product2/3
  Product2/1 -> Sum/2
  In/1 -> Integrator1/2, Sum1/1
  Sum1/1 -> Sum/1
  Integrator1/1 -> Out/1, Sum1/2
  Integrator/1 -> Product2/1, Product1/2
  Product1/1 -> Out_dot/1, Integrator1/1
  Wn/1 -> Product1/1, Product/1
  Sum/1 -> Product/2
  Product/1 -> Integrator/1

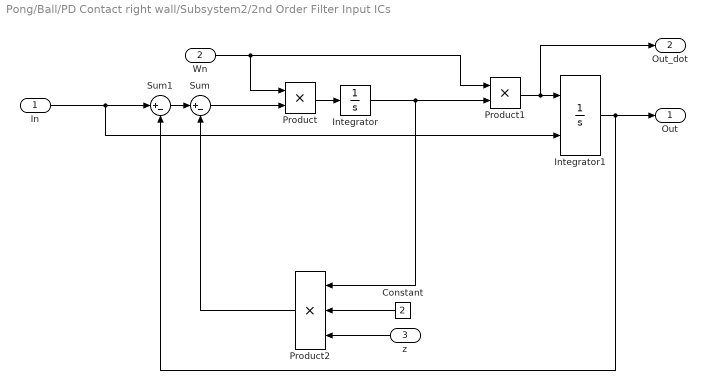
== system Pong/Ball/PD Contact right wall/Subsystem2/2nd Order Filter Input ICs ==
  In : Inport  OutDataType=sfix(16)  OutScaling=2^0
  Wn : Inport  Port=2  OutDataType=sfix(16)  OutScaling=2^0
  z : Inport  Orientation=left  Port=3  OutDataType=sfix(16)  OutScaling=2^0
  Constant : Constant  Orientation=left  Value=2  OutDataType=sfix(16)  OutScaling=2^0
  Integrator : Integrator
  Integrator1 : Integrator  InitialConditionSource=external
  Product : Product  OutDataType=sfix(16)  OutScaling=2^0  RndMeth=Zero
  Product1 : Product  OutDataType=sfix(16)  OutScaling=2^0  RndMeth=Zero
  Product2 : Product  Orientation=left  Inputs=3  OutDataType=sfix(16)  OutScaling=2^0  RndMeth=Zero
  Sum : Sum  Inputs=|+-  OutDataType=sfix(16)  OutScaling=2^0
  Sum1 : Sum  Inputs=|+-  OutDataType=sfix(16)  OutScaling=2^0
  Out : Outport  OutDataType=sfix(16)  OutScaling=2^0
  Out_dot : Outport  Port=2  OutDataType=sfix(16)  OutScaling=2^0
  wires:
  Constant/1 -> Product2/2
  z/1 -> Product2/3
  Product2/1 -> Sum/2
  In/1 -> Integrator1/2, Sum1/1
  Sum1/1 -> Sum/1
  Integrator1/1 -> Out/1, Sum1/2
  Integrator/1 -> Product2/1, Product1/2
  Product1/1 -> Out_dot/1, Integrator1/1
  Wn/1 -> Product1/1, Product/1
  Sum/1 -> Product/2
  Product/1 -> Integrator/1

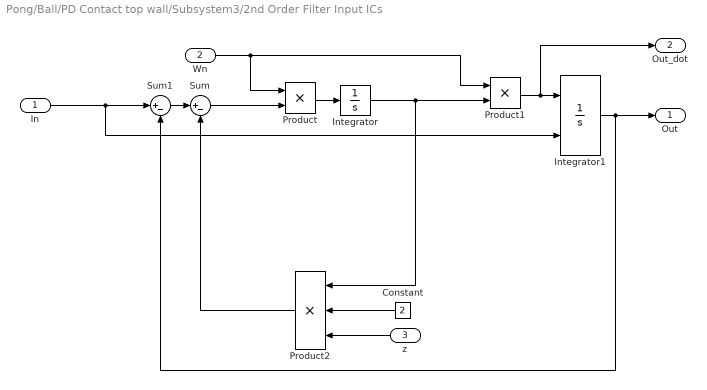
== system Pong/Ball/PD Contact top wall/Subsystem3/2nd Order Filter Input ICs ==
  In : Inport  OutDataType=sfix(16)  OutScaling=2^0
  Wn : Inport  Port=2  OutDataType=sfix(16)  OutScaling=2^0
  z : Inport  Orientation=left  Port=3  OutDataType=sfix(16)  OutScaling=2^0
  Constant : Constant  Orientation=left  Value=2  OutDataType=sfix(16)  OutScaling=2^0
  Integrator : Integrator
  Integrator1 : Integrator  InitialConditionSource=external
  Product : Product  OutDataType=sfix(16)  OutScaling=2^0  RndMeth=Zero
  Product1 : Product  OutDataType=sfix(16)  OutScaling=2^0  RndMeth=Zero
  Product2 : Product  Orientation=left  Inputs=3  OutDataType=sfix(16)  OutScaling=2^0  RndMeth=Zero
  Sum : Sum  Inputs=|+-  OutDataType=sfix(16)  OutScaling=2^0
  Sum1 : Sum  Inputs=|+-  OutDataType=sfix(16)  OutScaling=2^0
  Out : Outport  OutDataType=sfix(16)  OutScaling=2^0
  Out_dot : Outport  Port=2  OutDataType=sfix(16)  OutScaling=2^0
  wires:
  Constant/1 -> Product2/2
  z/1 -> Product2/3
  Product2/1 -> Sum/2
  In/1 -> Integrator1/2, Sum1/1
  Sum1/1 -> Sum/1
  Integrator1/1 -> Out/1, Sum1/2
  Integrator/1 -> Product2/1, Product1/2
  Product1/1 -> Out_dot/1, Integrator1/1
  Wn/1 -> Product1/1, Product/1
  Sum/1 -> Product/2
  Product/1 -> Integrator/1

== matlab function Omni/Torque to PWM/Smart Saturation ==
  data: u input inherited; y output inherited size=3
function y = fcn(u)
% Smart Saturation: allows channels to go up to 1.6A 
% unless the total exceeds 2.2A in which case all channels
% are scaled so that the cumulative current is equal to 2.2A.

y = zeros(3,1);
MAX_CURRENT = 2.2; % Define the maximum cumulative current here

total = sum(abs(u));
if (total > MAX_CURRENT)
    y = MAX_CURRENT/total*u;
else
    y = u;
end

== matlab function Omni/Torque to PWM/Joint Torque to Motor Torque ==
  data: t input inherited; y output inherited
function y = fcn( t)
% Smart Saturation: allows channels to go up to 1.6A 
% unless the total exceeds 2.2A in which case all channels
% are scaled so that the cumulative current is equal to 2.2A.
y=[0 0 0]'

y(1)=t(1);
y(3)=t(3);
y(2)=t(2)-t(3);


end

== matlab function Omni/Forward Kinematics  ==
  data: pos output inherited; q input inherited; Rot output inherited; tool_offset input inherited; Jac output inherited
function [pos,Rot,Jac]    = fcn(q,tool_offset)
% This block supports the Embedded MATLAB subset.
% See the help menu for details. 

% Link lengths
L1 = .132;
L2 = .132;

%Define A-matrices
%A1= DH(a_i ,alpha_i    ,d_i    ,theta_i)
A1 = DH(0   ,-pi()/2    ,0      ,q(1));
A2 = DH(L1  ,0          ,0      ,q(2));
A3 = DH(L2   ,0     ,0     ,q(3)-pi/2);

%Define T Matrices
T01=A1;
T02=T01*A2;
T03=T02*A3;

%Axes of rotation in base coordinates. 

z0=[0 0 1]';
z1=T01(1:3,3);
z2=T02(1:3,3);

%Coordinate Frame origins in Base frame coordinates

p0=[0 0 0]';
p1=T01(1:3,4);
p2=T02(1:3,4);
p3=T03(1:3,4);


%tool_offset given with respect to frame 3.
T_tool=T03*tool_offset;
Rot=T03(1:3,1:3);
pos=T_tool(1:3,4);

%Formulation of the Jacobian

%%%%%%%%%%%%%%%%%%%%%%%%%%%%JACOBIAN%%%%%%%%%%%%%%%%%%%%%%%%
Jac = [cross(z0,(pos-p0)) cross(z1,(pos-p1)) cross(z2,(pos-p2))
    z0 z1 z2];

end

function A = DH(a_x, alpha_x, d_z, theta_z)

A_R_z = [cos(theta_z) -sin(theta_z) 0 0;
         sin(theta_z) cos(theta_z) 0 0;
         0 0 1 0;
         0 0 0 1];

A_T_z = [1 0 0 0;
         0 1 0 0;
         0 0 1 d_z;
         0 0 0 1];
     
  

A_T_x = [1 0 0 a_x;
         0 1 0 0;
         0 0 1 0;
         0 0 0 1];

A_R_x = [1 0 0 0;
         0 cos(alpha_x) -sin(alpha_x)  0;
         0 sin(alpha_x) cos(alpha_x) 0;
         0 0 0 1];

A = A_R_z*A_T_z*A_T_x*A_R_x;

end

== matlab function Omni/Encoders to Joints q1, q2, q3/Embedded MATLAB Function ==
  data: m input inherited; q output inherited
function q = Motors_2_Joints(m)
q = m;
q(1) = m(1);
q(2) = m(2);
q(3) = m(3) - m(2) -pi/2;
end
